simulink model "modelo_q3"  (R2016a)
settings: Solver=VariableStepAuto  StartTime=0.0  StopTime=40  MaxStep=0.01  RelTol=1e-3
values from neighbouring files (symbols this model uses):
  A = double(subs(jacobian(f),[x1 x2],[0 0]))    [Projeto.m]    (also in q2.m = [0 1  0   0; questao2.m = [0 1 0 0; questao3.m = double(subs(jacobian(f,x),[x1 x2 x3 x4],[0 0 0 0])))
  B = double(subs(u, [x1 x2],[0 0]))    [Projeto.m]    (also in q2.m = [  0; questao2.m = [0; 1/M; 0; -1/(M*L)]; questao3.m = double(subs(jacobian(f,u),[x3 x4 u],[0 0 0])))
  C = [1 0 0 ... (first row only)    [Projeto.m]    (also in q2.m = [1 0 0 0]; questao2.m = [1 0 0 0]; questao3.m = [1 0 0 0])
  K = place(A,B,P1)    [Projeto.m]    (also in questao2.m = kb*T^-1; questao3.m = place(A,B, [pd pd-.01 pd+0.05 pd+0.02]))
  Km = Ka(:,5:7)    [questao2.m]    (also in questao3.m = Ka(1,5))
  Kx = Ka(1,1:4)    [questao3.m]
  Lk = Lk'    [questao3.m]
  x0 = [pi/180*30 0 0]    [Projeto.m]    (also in questao2.m = [0 0 pi/180*10 0]; questao3.m = [0 0 pi/180*20 0])
  x0obs = [pi/180*45 ; 0; 0]    [Projeto.m]    (also in questao2.m = [0 0 pi/180*10 0]; questao3.m = [0; 0; pi/180*20; 0])
settings Model: Creator=Regner  LastModifiedBy=Regner

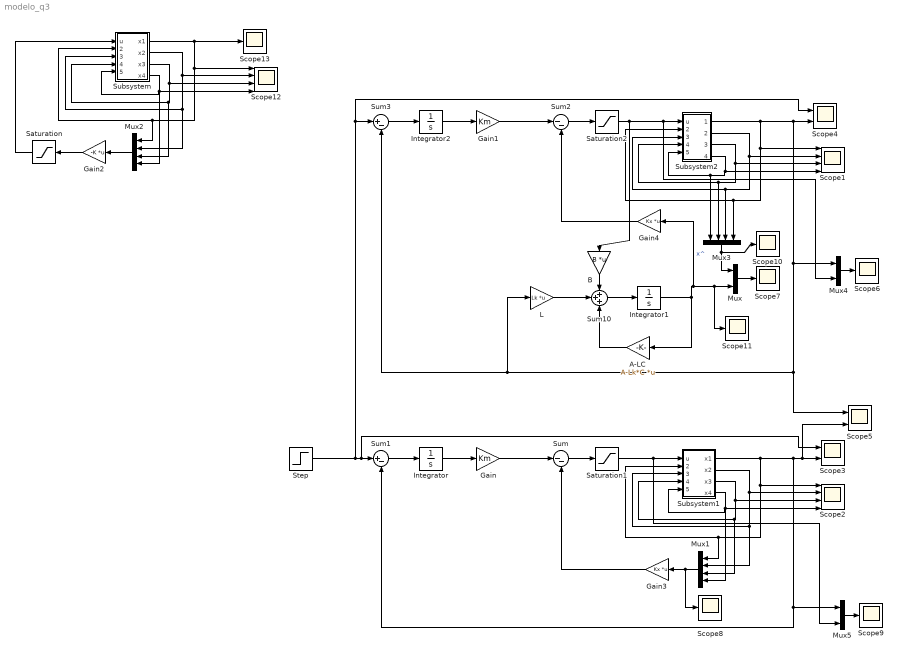
== system modelo_q3 ==
  A-LC : Gain  Gain=A-Lk*C  Multiplication=Matrix(K*u)
  B : Gain  Gain=B  Multiplication=Matrix(K*u)
  Gain : Gain  Gain=Km
  Gain1 : Gain  Gain=Km
  Gain2 : Gain  Gain=-K  Multiplication=Matrix(K*u)
  Gain3 : Gain  Gain=Kx  Multiplication=Matrix(K*u)
  Gain4 : Gain  Gain=Kx  Multiplication=Matrix(K*u)
  Integrator : Integrator
  Integrator1 : Integrator  InitialCondition=x0obs  ZeroCross=off
  Integrator2 : Integrator
  L : Gain  Gain=Lk  Multiplication=Matrix(K*u)
  Mux : Mux  Inputs=2
  Mux1 : Mux
  Mux2 : Mux
  Mux3 : Mux
  Mux4 : Mux  Inputs=2
  Mux5 : Mux  Inputs=2
  Saturation : Saturate  UpperLimit=50  LowerLimit=-50
  Saturation1 : Saturate  UpperLimit=50  LowerLimit=-50
  Saturation2 : Saturate  UpperLimit=50  LowerLimit=-50
  Scope1 : Scope  NumInputPorts=4
  Scope{6..11,13} (7 alike) : Scope
  Scope12 : Scope  NumInputPorts=4
  Scope2 : Scope  NumInputPorts=4
  Scope3 : Scope  NumInputPorts=2
  Scope4 : Scope  NumInputPorts=2
  Scope5 : Scope  NumInputPorts=2
  Step : Step  Time=20  After=pi/180*0  SampleTime=0
  Subsystem : Subsystem
  Subsystem1 : Subsystem
  Subsystem2 : Subsystem
  Sum : Sum  Inputs=|--
  Sum1 : Sum  Inputs=|+-
  Sum10 : Sum  Inputs=+++
  Sum2 : Sum  Inputs=|--
  Sum3 : Sum  Inputs=|+-
  wires:
  Sum10/1 -> Integrator1/1
  L/1 -> Sum10/2
  A-LC/1 -> Sum10/3
  Integrator1/1 -> Gain4/1, Scope11/1, Mux/2, A-LC/1  "x^"
  B/1 -> Sum10/1
  Mux/1 -> Scope7/1
  Mux2/1 -> Gain2/1
  Gain2/1 -> Saturation/1
  Subsystem/4(x4) -> Mux2/4, Scope12/4, Subsystem/5(x4e)
  Subsystem/3(x3) -> Mux2/3, Subsystem/4(x3e), Scope12/3
  Subsystem/2(x2) -> Mux2/2, Subsystem/3(x2e), Scope12/2
  Saturation/1 -> Subsystem/1(u)
  Subsystem/1(x1) -> Scope13/1, Mux2/1, Subsystem/2(x1e), Scope12/1
  Mux1/1 -> Scope8/1, Gain3/1
  Subsystem1/4(x4) -> Subsystem1/5(x4e), Scope2/4, Mux1/4
  Subsystem1/3(x3) -> Scope2/3, Subsystem1/4(x3e), Mux1/3
  Subsystem1/2(x2) -> Scope2/2, Subsystem1/3(x2e), Mux1/2
  Gain3/1 -> Sum/2
  Sum/1 -> Saturation1/1
  Gain/1 -> Sum/1
  Integrator/1 -> Gain/1
  Sum1/1 -> Integrator/1
  Subsystem2/4(x4) -> Scope1/4, Mux3/1, Subsystem2/5(x4e)
  Subsystem2/3(x3) -> Mux3/2, Subsystem2/4(x3e), Scope1/3
  Subsystem2/2(x2) -> Mux3/3, Subsystem2/3(x2e), Scope1/2
  Subsystem2/1(x1) -> Scope4/2, Mux4/1, L/1, Sum3/2, Scope5/1, Mux3/4, Subsystem2/2(x1e), Scope1/1
  Sum2/1 -> Saturation2/1
  Gain1/1 -> Sum2/1
  Integrator2/1 -> Gain1/1
  Sum3/1 -> Integrator2/1
  Step/1 -> Scope4/1, Sum3/1, Scope3/1, Sum1/1
  Saturation2/1 -> B/1, Mux4/2, Subsystem2/1(u)
  Gain4/1 -> Sum2/2
  Mux3/1 -> Scope10/1, Mux/1
  Mux4/1 -> Scope6/1
  Subsystem1/1(x1) -> Scope2/1, Subsystem1/2(x1e), Mux1/1, Scope5/2, Scope3/2, Mux5/1, Sum1/2
  Saturation1/1 -> Mux5/2, Subsystem1/1(u)
  Mux5/1 -> Scope9/1

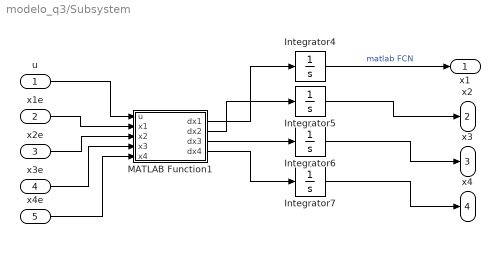
== system modelo_q3/Subsystem ==
  u : Inport
  x1e : Inport  Port=2
  x2e : Inport  Port=3
  x3e : Inport  Port=4
  x4e : Inport  Port=5
  Integrator4 : Integrator  ZeroCross=off
  Integrator5 : Integrator  ZeroCross=off
  Integrator6 : Integrator  InitialCondition=0.1  ZeroCross=off
  Integrator7 : Integrator  ZeroCross=off
  MATLAB Function1 : MATLAB Function  TreatAsAtomicUnit=on
  x1 : Outport
  x2 : Outport  Port=2
  x3 : Outport  Port=3
  x4 : Outport  Port=4
  wires:
  x2e/1 -> MATLAB Function1/3(x2)
  x4e/1 -> MATLAB Function1/5(x4)
  x3e/1 -> MATLAB Function1/4(x3)
  x1e/1 -> MATLAB Function1/2(x1)
  Integrator5/1 -> x2/1
  Integrator7/1 -> x4/1
  u/1 -> MATLAB Function1/1(u)
  MATLAB Function1/4(dx4) -> Integrator7/1
  MATLAB Function1/1(dx1) -> Integrator4/1
  Integrator4/1 -> x1/1  "matlab FCN"
  MATLAB Function1/3(dx3) -> Integrator6/1
  MATLAB Function1/2(dx2) -> Integrator5/1
  Integrator6/1 -> x3/1

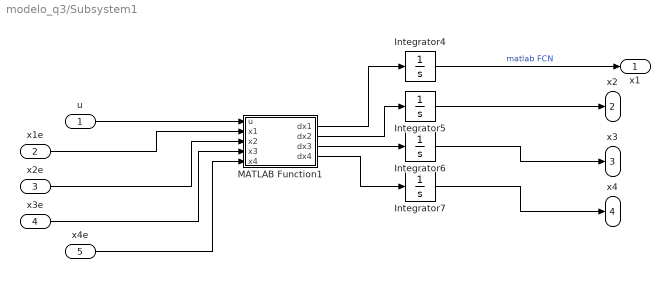
== system modelo_q3/Subsystem1 ==
  u : Inport
  x1e : Inport  Port=2
  x2e : Inport  Port=3
  x3e : Inport  Port=4
  x4e : Inport  Port=5
  Integrator4 : Integrator  InitialCondition=x0(1)  ZeroCross=off
  Integrator5 : Integrator  InitialCondition=x0(2)  ZeroCross=off
  Integrator6 : Integrator  InitialCondition=x0(3)  ZeroCross=off
  Integrator7 : Integrator  InitialCondition=x0(4)  ZeroCross=off
  MATLAB Function1 : MATLAB Function  TreatAsAtomicUnit=on
  x1 : Outport
  x2 : Outport  Port=2
  x3 : Outport  Port=3
  x4 : Outport  Port=4
  wires:
  Integrator6/1 -> x3/1
  MATLAB Function1/2(dx2) -> Integrator5/1
  MATLAB Function1/3(dx3) -> Integrator6/1
  Integrator4/1 -> x1/1  "matlab FCN"
  MATLAB Function1/1(dx1) -> Integrator4/1
  MATLAB Function1/4(dx4) -> Integrator7/1
  u/1 -> MATLAB Function1/1(u)
  Integrator7/1 -> x4/1
  Integrator5/1 -> x2/1
  x1e/1 -> MATLAB Function1/2(x1)
  x3e/1 -> MATLAB Function1/4(x3)
  x4e/1 -> MATLAB Function1/5(x4)
  x2e/1 -> MATLAB Function1/3(x2)

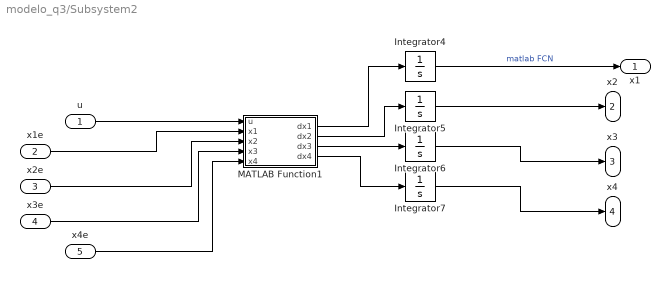
== system modelo_q3/Subsystem2 ==
  u : Inport
  x1e : Inport  Port=2
  x2e : Inport  Port=3
  x3e : Inport  Port=4
  x4e : Inport  Port=5
  Integrator4 : Integrator  InitialCondition=x0(1)  ZeroCross=off
  Integrator5 : Integrator  InitialCondition=x0(2)  ZeroCross=off
  Integrator6 : Integrator  InitialCondition=x0(3)  ZeroCross=off
  Integrator7 : Integrator  InitialCondition=x0(4)  ZeroCross=off
  MATLAB Function1 : MATLAB Function  TreatAsAtomicUnit=on
  x1 : Outport
  x2 : Outport  Port=2
  x3 : Outport  Port=3
  x4 : Outport  Port=4
  wires:
  x2e/1 -> MATLAB Function1/3(x2)
  x4e/1 -> MATLAB Function1/5(x4)
  x3e/1 -> MATLAB Function1/4(x3)
  x1e/1 -> MATLAB Function1/2(x1)
  Integrator5/1 -> x2/1
  Integrator7/1 -> x4/1
  u/1 -> MATLAB Function1/1(u)
  MATLAB Function1/4(dx4) -> Integrator7/1
  MATLAB Function1/1(dx1) -> Integrator4/1
  Integrator4/1 -> x1/1  "matlab FCN"
  MATLAB Function1/3(dx3) -> Integrator6/1
  MATLAB Function1/2(dx2) -> Integrator5/1
  Integrator6/1 -> x3/1

== matlab function modelo_q3/Subsystem/MATLAB Function1 ==
  data: dx1 output; dx2 output; dx3 output; u input; x1 input; x2 input; x3 input; x4 input; dx4 output
function [dx1,dx2,dx3,dx4] = fcn(u, x1, x2, x3, x4)
%#codegen
M = 1;
L = 1;
m = 0.5;
g = 9.81;


dx1 = x2;
dx2 = (u-m*g*sin(x3)*cos(x3)+m*L*x4^2*sin(x3))/(M+m-m*cos(x3)^2);
dx3 = x4;
f4_num = m*g*sin(x3)-((u+m*L*x4^2*sin(x3))*m*cos(x3))/(M+m);
f4_den = m*L-(m^2*L*cos(x3)^2)/(M+m);
dx4 = f4_num/f4_den;
end

== matlab function modelo_q3/Subsystem1/MATLAB Function1 ==
  data: dx1 output; dx2 output; dx3 output; u input; x1 input; x2 input; x3 input; x4 input; dx4 output
function [dx1,dx2,dx3,dx4] = fcn(u, x1, x2, x3, x4)
%#codegen
M = 1;
L = 1;
m = 0.5;
g = 9.81;


dx1 = x2;
dx2 = (u-m*g*sin(x3)*cos(x3)+m*L*x4^2*sin(x3))/(M+m-m*cos(x3)^2);
dx3 = x4;
f4_num = m*g*sin(x3)-((u+m*L*x4^2*sin(x3))*m*cos(x3))/(M+m);
f4_den = m*L-(m^2*L*cos(x3)^2)/(M+m);
dx4 = f4_num/f4_den;
end

== matlab function modelo_q3/Subsystem2/MATLAB Function1 ==
  data: dx1 output; dx2 output; dx3 output; u input; x1 input; x2 input; x3 input; x4 input; dx4 output
function [dx1,dx2,dx3,dx4] = fcn(u, x1, x2, x3, x4)
%#codegen
M = 1;
L = 1;
m = 0.5;
g = 9.81;


dx1 = x2;
dx2 = (u-m*g*sin(x3)*cos(x3)+m*L*x4^2*sin(x3))/(M+m-m*cos(x3)^2);
dx3 = x4;
f4_num = m*g*sin(x3)-((u+m*L*x4^2*sin(x3))*m*cos(x3))/(M+m);
f4_den = m*L-(m^2*L*cos(x3)^2)/(M+m);
dx4 = f4_num/f4_den;
end
